simulink subsystem "s3DOF_to_6DOF"  (R2023b)
settings: Solver=VariableStepAuto  StartTime=0.0  StopTime=10.0  RelTol=1e-3
undefined symbols (not defined in the file): alt0, heading0, inertia, theta0, V0, wy0
libraries: aerolibtransform2 x2, aerolibasang x1, sharedtransform x1
settings Model: Creator=szdaniel  LastModifiedBy=szdaniel

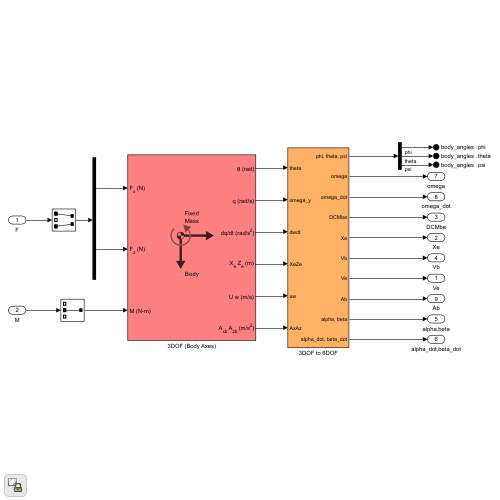
[thumbnail: Simulink's stored preview of the top-level diagram]
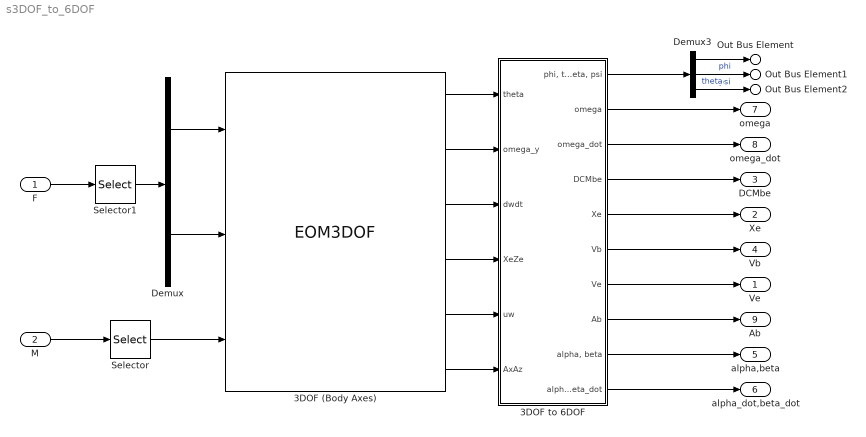
== system s3DOF_to_6DOF ==
  F : Inport
  M : Inport  Port=2
  3DOF (Body Axes) : EOM3DOF  v_ini=V0  theta_ini=theta0  q_ini=wy0  alpha_ini=alpha0  pos_ini=[0 -alt0]  mass=mass  Iyy=inertia(2,2)  g=0  mdot_flag=off
  3DOF to 6DOF : Subsystem
  Demux : Demux  Outputs=2
  Demux3 : Demux  Outputs=3
  Selector : Selector  IndexMode=Zero-based  InputPortWidth=3  IndexOptions=Index vector (dialog)  Indices=1  OutputSizes=1
  Selector1 : Selector  IndexMode=Zero-based  InputPortWidth=3  IndexOptions=Index vector (dialog)  Indices=[0 2]  OutputSizes=1
  Ve : Outport  Unit=m/s  VectorParamsAs1DForOutWhenUnconnected=off
  Xe : Outport  Port=2  Unit=m  VectorParamsAs1DForOutWhenUnconnected=off
  DCMbe : Outport  Port=3  VectorParamsAs1DForOutWhenUnconnected=off
  Vb : Outport  Port=4  Unit=m/s  VectorParamsAs1DForOutWhenUnconnected=off
  alpha,beta : Outport  Port=5  Unit=rad  VectorParamsAs1DForOutWhenUnconnected=off
  alpha_dot,beta_dot : Outport  Port=6  Unit=rad/s  VectorParamsAs1DForOutWhenUnconnected=off
  omega : Outport  Port=7  Unit=rad/s  VectorParamsAs1DForOutWhenUnconnected=off
  omega_dot : Outport  Port=8  Unit=rad/s^2  VectorParamsAs1DForOutWhenUnconnected=off
  Ab : Outport  Port=9  Unit=m/s^2  VectorParamsAs1DForOutWhenUnconnected=off
  Out Bus Element : Outport  Port=10  PortName=body_angles  Element=phi
  Out Bus Element1 : Outport  Port=10  PortName=body_angles  Element=theta
  Out Bus Element2 : Outport  Port=10  PortName=body_angles  Element=psi
  wires:
  3DOF (Body Axes)/1 -> 3DOF to 6DOF/1(theta)
  Selector/1 -> 3DOF (Body Axes)/3
  Selector1/1 -> Demux/1
  3DOF to 6DOF/2(omega) -> omega/1
  3DOF to 6DOF/3(omega_dot) -> omega_dot/1
  3DOF to 6DOF/5(Xe) -> Xe/1
  3DOF to 6DOF/7(Ve) -> Ve/1
  3DOF to 6DOF/10("alpha_dot, beta_dot") -> alpha_dot,beta_dot/1
  3DOF (Body Axes)/2 -> 3DOF to 6DOF/2(omega_y)
  3DOF to 6DOF/6(Vb) -> Vb/1
  3DOF to 6DOF/8(Ab) -> Ab/1
  3DOF to 6DOF/9("alpha, beta") -> alpha,beta/1
  3DOF to 6DOF/4(DCMbe) -> DCMbe/1
  3DOF (Body Axes)/3 -> 3DOF to 6DOF/3(dwdt)
  3DOF (Body Axes)/4 -> 3DOF to 6DOF/4(XeZe)
  3DOF (Body Axes)/5 -> 3DOF to 6DOF/5(uw)
  3DOF (Body Axes)/6 -> 3DOF to 6DOF/6(AxAz)
  Demux/1 -> 3DOF (Body Axes)/1
  Demux/2 -> 3DOF (Body Axes)/2
  F/1 -> Selector1/1
  M/1 -> Selector/1
  Demux3/3 -> Out Bus Element2/1  "psi"
  3DOF to 6DOF/1("phi, theta, psi") -> Demux3/1
  Demux3/1 -> Out Bus Element/1  "phi"
  Demux3/2 -> Out Bus Element1/1  "theta"

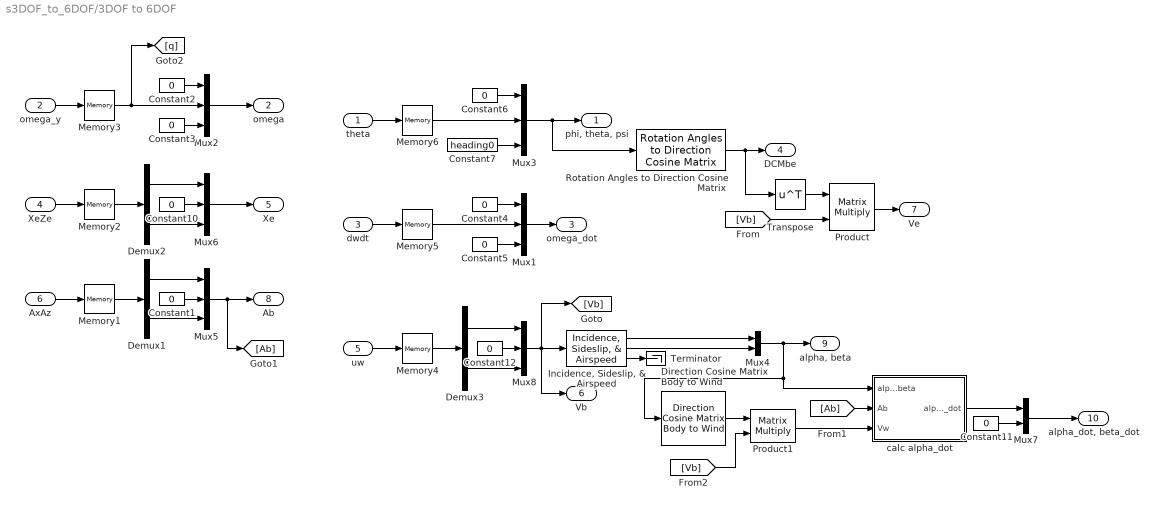
== system s3DOF_to_6DOF/3DOF to 6DOF ==
  theta : Inport
  omega_y : Inport  Port=2
  dwdt : Inport  Port=3
  XeZe : Inport  Port=4
  uw : Inport  Port=5
  AxAz : Inport  Port=6
  Constant{1..6,10..12} (9 alike) : Constant  Value=0
  Constant7 : Constant  Value=heading0
  Demux1 : Demux  Outputs=2
  Demux2 : Demux  Outputs=2
  Demux3 : Demux  Outputs=2
  Direction Cosine Matrix Body to Wind : aerolibtransform2/Direction Cosine Matrix Body to Wind
  "Incidence, Sideslip, & Airspeed" : aerolibasang/Incidence, Sideslip, & Airspeed
  Memory1 : Memory
  Memory2 : Memory  InitialCondition=[0 -alt0]
  Memory3 : Memory  InitialCondition=wy0
  Memory4 : Memory  InitialCondition=[V0 0]
  Memory5 : Memory
  Memory6 : Memory  InitialCondition=theta0
  Mux{1..3,5..6,8} (6 alike) : Mux  Inputs=3
  Mux4 : Mux  Inputs=2
  Mux7 : Mux  Inputs=2
  Product : Product  Multiplication=Matrix(*)  InputSameDT=on  SaturateOnIntegerOverflow=on  OutDataTypeStr=Inherit: Same as first input
  Product1 : Product  Multiplication=Matrix(*)  InputSameDT=on  SaturateOnIntegerOverflow=on  OutDataTypeStr=Inherit: Same as first input
  Rotation Angles to Direction Cosine Matrix : sharedtransform/Rotation Angles to Direction Cosine Matrix  rotationOrder=ZYX  aMode=aMode
  Terminator : Terminator
  Transpose : Math  Operator=transpose  SignedPower=on
  calc alpha_dot : Subsystem
  "phi, theta, psi" : Outport  Unit=rad  VectorParamsAs1DForOutWhenUnconnected=off
  omega : Outport  Port=2  Unit=rad/s  VectorParamsAs1DForOutWhenUnconnected=off
  omega_dot : Outport  Port=3  Unit=rad/s^2  VectorParamsAs1DForOutWhenUnconnected=off
  DCMbe : Outport  Port=4  VectorParamsAs1DForOutWhenUnconnected=off
  Xe : Outport  Port=5  Unit=m  VectorParamsAs1DForOutWhenUnconnected=off
  Vb : Outport  Port=6  Unit=m/s  VectorParamsAs1DForOutWhenUnconnected=off
  Ve : Outport  Port=7  Unit=m/s  VectorParamsAs1DForOutWhenUnconnected=off
  Ab : Outport  Port=8  Unit=m/s^2  VectorParamsAs1DForOutWhenUnconnected=off
  "alpha, beta" : Outport  Port=9  Unit=rad  VectorParamsAs1DForOutWhenUnconnected=off
  "alpha_dot, beta_dot" : Outport  Port=10  Unit=rad/s  VectorParamsAs1DForOutWhenUnconnected=off
  wires:
  Memory6/1 -> Mux3/2
  theta/1 -> Memory6/1
  Memory5/1 -> Mux1/2
  dwdt/1 -> Memory5/1
  Memory4/1 -> Demux3/1
  uw/1 -> Memory4/1
  Memory3/1 -> Mux2/2, [q]
  omega_y/1 -> Memory3/1
  XeZe/1 -> Memory2/1
  Memory2/1 -> Demux2/1
  AxAz/1 -> Memory1/1
  Memory1/1 -> Demux1/1
  Mux7/1 -> "alpha_dot, beta_dot"/1
  Constant5/1 -> Mux1/3
  Rotation Angles to Direction Cosine Matrix/1 -> Transpose/1, DCMbe/1
  Mux8/1 -> [Vb], "Incidence, Sideslip, & Airspeed"/1, Vb/1
  Product/1 -> Ve/1
  Mux6/1 -> Xe/1
  Mux1/1 -> omega_dot/1
  Mux2/1 -> omega/1
  "Incidence, Sideslip, & Airspeed"/3 -> Terminator/1
  "Incidence, Sideslip, & Airspeed"/1 -> Mux4/1
  Product1/1 -> calc alpha_dot/3(Vw)
  Direction Cosine Matrix Body to Wind/1 -> Product1/1
  Demux3/1 -> Mux8/1
  Constant12/1 -> Mux8/2
  Demux3/2 -> Mux8/3
  Constant11/1 -> Mux7/2
  [Vb] -> Product1/2
  [Ab] -> calc alpha_dot/2(Ab)
  calc alpha_dot/1(alpha_dot) -> Mux7/1
  [Vb] -> Product/2
  Transpose/1 -> Product/1
  Constant10/1 -> Mux6/2
  Demux2/2 -> Mux6/3
  Demux2/1 -> Mux6/1
  "Incidence, Sideslip, & Airspeed"/2 -> Mux4/2
  Mux4/1 -> calc alpha_dot/1(alpha,beta), Direction Cosine Matrix Body to Wind/1, "alpha, beta"/1
  Mux3/1 -> Rotation Angles to Direction Cosine Matrix/1, "phi, theta, psi"/1
  Constant7/1 -> Mux3/3
  Constant6/1 -> Mux3/1
  Constant4/1 -> Mux1/1
  Constant3/1 -> Mux2/3
  Constant2/1 -> Mux2/1
  Constant1/1 -> Mux5/2
  Demux1/2 -> Mux5/3
  Demux1/1 -> Mux5/1
  Mux5/1 -> [Ab], Ab/1

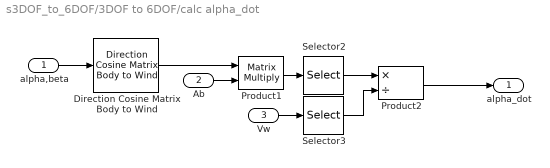
== system s3DOF_to_6DOF/3DOF to 6DOF/calc alpha_dot ==
  alpha,beta : Inport
  Ab : Inport  Port=2
  Vw : Inport  Port=3
  Direction Cosine Matrix Body to Wind : aerolibtransform2/Direction Cosine Matrix Body to Wind
  Product1 : Product  Multiplication=Matrix(*)  InputSameDT=on  SaturateOnIntegerOverflow=on  OutDataTypeStr=Inherit: Same as first input
  Product2 : Product  Inputs=*/  InputSameDT=on  SaturateOnIntegerOverflow=on  OutDataTypeStr=Inherit: Same as first input
  Selector2 : Selector  IndexMode=Zero-based  InputPortWidth=3  IndexOptions=Index vector (dialog)  Indices=2  OutputSizes=1
  Selector3 : Selector  IndexMode=Zero-based  InputPortWidth=3  IndexOptions=Index vector (dialog)  Indices=0  OutputSizes=1
  alpha_dot : Outport  VectorParamsAs1DForOutWhenUnconnected=off
  wires:
  Vw/1 -> Selector3/1
  Ab/1 -> Product1/2
  Product2/1 -> alpha_dot/1
  alpha,beta/1 -> Direction Cosine Matrix Body to Wind/1
  Selector3/1 -> Product2/2
  Selector2/1 -> Product2/1
  Product1/1 -> Selector2/1
  Direction Cosine Matrix Body to Wind/1 -> Product1/1
